simulink model "Simulink_asserv_Disc_21Mars_V2023b"  (R2023b)
settings: Solver=ode45  StartTime=0.0  StopTime=2500  FixedStep=0.01  RelTol=1e-3
model workspace (MAT data in the model file):
  AmbiantTemp = 23
  CondSig_mesureTemp_Gain = 3.3
  CondSig_mesureTemp_Vsub = 1.85
  DivTen_mesureTemp_R_pullup = 10000
  DivTen_mesureTemp_Vcc = 5
  Estimateur_alpha = 0.5
  Filtre_mesureTemp_deno = [0.0033 1]
  Gain_Comparateur_VoltageControle = 0.32
  RC_deno = [3.22e-08 3.04e-05 0.00955 1]
  Sig = Simulink.Signal
  Sig.DataType = 'auto'
  Sig.Dimensions = -1
  Sig.DimensionsMode = 'auto'
  Sig.Complexity = 'auto'
  Sig.SampleTime = -1
  Sig.SamplingMode = 'auto'
  SourceCourant_Gain_Vcontrole_vers_A = 3.1564
  ThermoRes_SHTEMP_A = 0.003354
  ThermoRes_SHTEMP_B = 0.00026
  ThermoRes_SHTEMP_C = 1.6e-06
  ThermoRes_SHTEMP_D = 6.3e-08
  ThermoRes_SH_A = -14.65719
  ThermoRes_SH_B = 4798.842
  ThermoRes_SH_C = -115334
  ThermoRes_SH_D = -3730535
  ThermoRes_SH_R_nom = 10000
  periodeEchant = 2
  periodeEchant_temp = 0.5
  setupDelay = 4
libraries: simulink x1
settings Model: SimulationMode=rapid-accelerator  Creator=alcot161  LastModifiedBy=alcot161
settings RTWCC: GPUComputeCapability=5.0

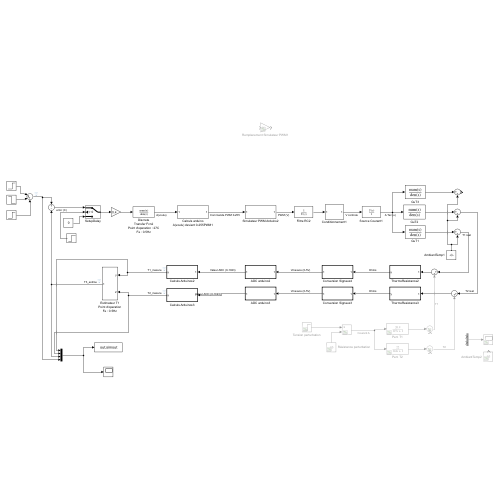
[thumbnail: Simulink's stored preview of the top-level diagram]
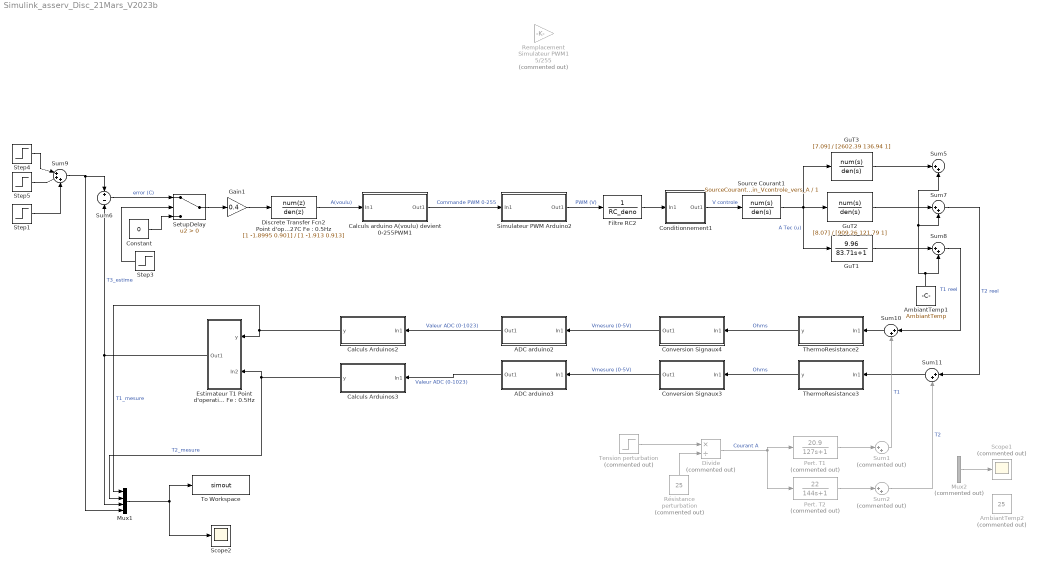
== system Simulink_asserv_Disc_21Mars_V2023b ==
  ADC arduino2 : Subsystem  TreatAsAtomicUnit=on
  ADC arduino3 : Subsystem  TreatAsAtomicUnit=on
  AmbiantTemp1 : Constant  Value=AmbiantTemp
  AmbiantTemp2 : Constant  Commented=on  Value=25
  Calculs Arduinos2 : Subsystem  TreatAsAtomicUnit=on
  Calculs Arduinos3 : Subsystem  TreatAsAtomicUnit=on
  Calculs arduino A(voulu) devient 0-255PWM1 : Subsystem
  Conditionnement1 : Subsystem
  Constant : Constant  Value=0  SampleTime=periodeEchant
  Conversion Signaux3 : Subsystem  TreatAsAtomicUnit=on
  Conversion Signaux4 : Subsystem  TreatAsAtomicUnit=on
  "Discrete Transfer Fcn2 Point d'operation : 27C Fe : 0.5Hz" : DiscreteTransferFcn  Numerator=[1 -1.8995 0.901]  Denominator=[1 -1.913 0.913]
  Divide : Product  Commented=on  Inputs=*/
  "Estimateur T1 Point d'operation Fe : 0.5Hz" : Subsystem
  Filtre RC2 : TransferFcn  Denominator=RC_deno
  Gain1 : Gain  Gain=0.4
  GuT1 : TransferFcn  Numerator=[9.96]  Denominator=[83.71 1]
  GuT2 : TransferFcn  Numerator=[8.07]  Denominator=[909.26 121.79 1]
  GuT3 : TransferFcn  Numerator=[7.09]  Denominator=[2602.39 136.94 1]
  Mux1 : Mux
  Mux2 : Mux  Commented=on  Inputs=2
  Pert. T1 : TransferFcn  Commented=on  Numerator=[20.9]  Denominator=[127 1]
  Pert. T2 : TransferFcn  Commented=on  Numerator=[22]  Denominator=[144 1]
  Remplacement Simulateur PWM1 : Gain  Commented=on  Gain=5/255
  Résistance perturbation : Constant  Commented=on  Value=25
  Scope1 : Scope  Commented=on
  Scope2 : Scope
  SetupDelay : Switch  Criteria=u2 > Threshold  SaturateOnIntegerOverflow=off  InputSameDT=off
  Simulateur PWM Arduino2 : Subsystem
  Source Courant1 : TransferFcn  Numerator=SourceCourant_Gain_Vcontrole_vers_A  Denominator=1
  Step1 : Step  Time=2130  After=3  SampleTime=0.05
  Step3 : Step  Time=setupDelay+1  SampleTime=periodeEchant
  Step4 : Step  Time=640  Before=AmbiantTemp  After=30  SampleTime=0.05
  Step5 : Step  Time=1290  After=-10  SampleTime=0.05
  Sum1 : Sum  Commented=on  Inputs=|++
  Sum{5,7..8,10..11} (5 alike) : Sum  Inputs=|++
  Sum2 : Sum  Commented=on  Inputs=|++
  Sum6 : Sum  Inputs=+|-  SampleTime=periodeEchant
  Sum9 : Sum  Inputs=|+++
  Tension perturbation : Step  Commented=on  Time=500  After=5  SampleTime=0.05
  ThermoResistance2 : Subsystem  TreatAsAtomicUnit=on
  ThermoResistance3 : Subsystem  TreatAsAtomicUnit=on
  To Workspace : ToWorkspace  VariableName=simout  SaveFormat=Timeseries  SampleTime=-1
  wires:
  ThermoResistance3/1(y) -> Conversion Signaux3/1(In1)  "Ohms"
  Step4/1 -> Sum9/1
  GuT2/1 -> Sum7/1
  Conversion Signaux3/1(Out1) -> ADC arduino3/1(In1)  "Vmesure (0-5V)"
  Sum9/1 -> Mux1/4, Sum6/1
  ADC arduino3/1(Out1) -> Calculs Arduinos3/1(In1)  "Valeur ADC (0-1023)"
  Simulateur PWM Arduino2/1(Out1) -> Filtre RC2/1  "PWM (V)"
  Step5/1 -> Sum9/2
  Conversion Signaux4/1(Out1) -> ADC arduino2/1(In1)  "Vmesure (0-5V)"
  AmbiantTemp1/1 -> Sum5/2, Sum7/2, Sum8/2
  Filtre RC2/1 -> Conditionnement1/1(In1)
  Calculs Arduinos2/1(y) -> Mux1/1, "Estimateur T1 Point d'operation Fe : 0.5Hz"/1(y)  "T1_mesure"
  ADC arduino2/1(Out1) -> Calculs Arduinos2/1(In1)  "Valeur ADC (0-1023)"
  Calculs arduino A(voulu) devient 0-255PWM1/1(Out1) -> Simulateur PWM Arduino2/1(In1)  "Commande PWM 0-255"
  Calculs Arduinos3/1(y) -> Mux1/2, "Estimateur T1 Point d'operation Fe : 0.5Hz"/2(In2)  "T2_mesure"
  Source Courant1/1 -> GuT3/1, GuT2/1, GuT1/1  "A Tec (u)"
  ThermoResistance2/1(y) -> Conversion Signaux4/1(In1)  "Ohms"
  Sum7/1 -> Sum11/1  "T2 reel"
  Conditionnement1/1(Out1) -> Source Courant1/1  "V controle"
  GuT1/1 -> Sum8/1
  GuT3/1 -> Sum5/1
  "Discrete Transfer Fcn2 Point d'operation : 27C Fe : 0.5Hz"/1 -> Calculs arduino A(voulu) devient 0-255PWM1/1(In1)  "A(voulu)"
  "Estimateur T1 Point d'operation Fe : 0.5Hz"/1(Out1) -> Mux1/3, Sum6/2  "T3_estime"
  Step3/1 -> SetupDelay/2
  Gain1/1 -> "Discrete Transfer Fcn2 Point d'operation : 27C Fe : 0.5Hz"/1
  Sum6/1 -> SetupDelay/1  "error (C)"
  SetupDelay/1 -> Gain1/1
  Constant/1 -> SetupDelay/3
  Sum8/1 -> Sum10/1  "T1 reel"
  Sum10/1 -> ThermoResistance2/1(In1)
  Sum11/1 -> ThermoResistance3/1(In1)
  Step1/1 -> Sum9/3
  Résistance perturbation/1 -> Divide/2
  Tension perturbation/1 -> Divide/1
  Divide/1 -> Pert. T2/1, Pert. T1/1  "Courant A"
  Sum1/1 -> Sum10/2  "T1"
  Sum2/1 -> Sum11/2  "T2"
  Pert. T1/1 -> Sum1/1
  Pert. T2/1 -> Sum2/1
  Mux2/1 -> Scope1/1
  Mux1/1 -> To Workspace/1, Scope2/1

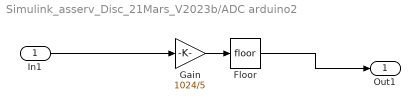
== system Simulink_asserv_Disc_21Mars_V2023b/ADC arduino2 ==
  In1 : Inport
  Floor : Rounding
  Gain : Gain  Gain=1024/5
  Out1 : Outport  SampleTime=periodeEchant_temp
  wires:
  In1/1 -> Gain/1
  Gain/1 -> Floor/1
  Floor/1 -> Out1/1

== system Simulink_asserv_Disc_21Mars_V2023b/ADC arduino3 ==
  In1 : Inport
  Floor : Rounding
  Gain : Gain  Gain=1024/5
  Out1 : Outport  SampleTime=periodeEchant_temp
  wires:
  In1/1 -> Gain/1
  Gain/1 -> Floor/1
  Floor/1 -> Out1/1

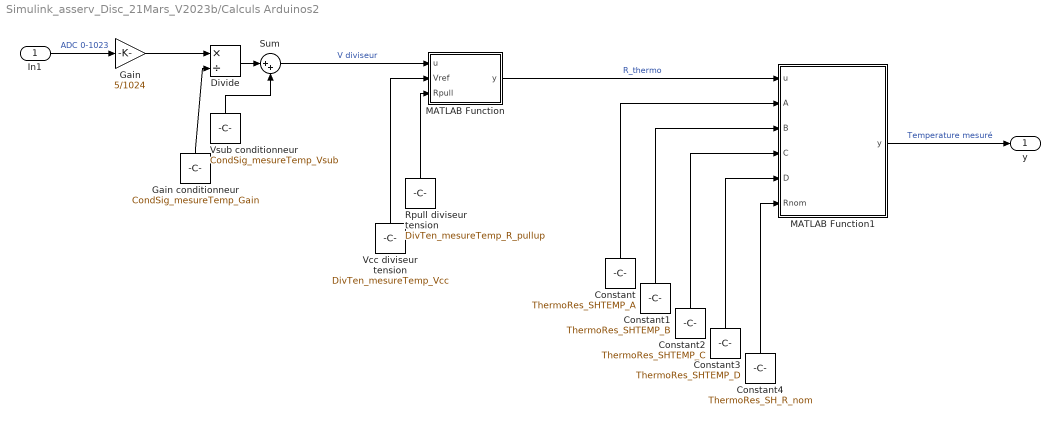
== system Simulink_asserv_Disc_21Mars_V2023b/Calculs Arduinos2 ==
  In1 : Inport
  Constant : Constant  Value=ThermoRes_SHTEMP_A
  Constant1 : Constant  Value=ThermoRes_SHTEMP_B
  Constant2 : Constant  Value=ThermoRes_SHTEMP_C
  Constant3 : Constant  Value=ThermoRes_SHTEMP_D
  Constant4 : Constant  Value=ThermoRes_SH_R_nom
  Divide : Product  Inputs=*/
  Gain : Gain  Gain=5/1024
  Gain conditionneur : Constant  Value=CondSig_mesureTemp_Gain
  MATLAB Function : MATLAB Function  TreatAsAtomicUnit=on
  MATLAB Function1 : MATLAB Function  TreatAsAtomicUnit=on
  Rpull diviseur tension : Constant  Value=DivTen_mesureTemp_R_pullup
  Sum : Sum  Inputs=|++
  Vcc diviseur tension : Constant  Value=DivTen_mesureTemp_Vcc
  Vsub conditionneur : Constant  Value=CondSig_mesureTemp_Vsub
  y : Outport
  wires:
  In1/1 -> Gain/1  "ADC 0-1023"
  Gain/1 -> Divide/1
  Gain conditionneur/1 -> Divide/2
  Divide/1 -> Sum/1
  Vsub conditionneur/1 -> Sum/2
  Sum/1 -> MATLAB Function/1(u)  "V diviseur"
  Rpull diviseur tension/1 -> MATLAB Function/3(Rpull)
  Vcc diviseur tension/1 -> MATLAB Function/2(Vref)
  MATLAB Function/1(y) -> MATLAB Function1/1(u)  "R_thermo"
  Constant/1 -> MATLAB Function1/2(A)
  Constant1/1 -> MATLAB Function1/3(B)
  Constant2/1 -> MATLAB Function1/4(C)
  Constant3/1 -> MATLAB Function1/5(D)
  Constant4/1 -> MATLAB Function1/6(Rnom)
  MATLAB Function1/1(y) -> y/1  "Temperature mesuré"

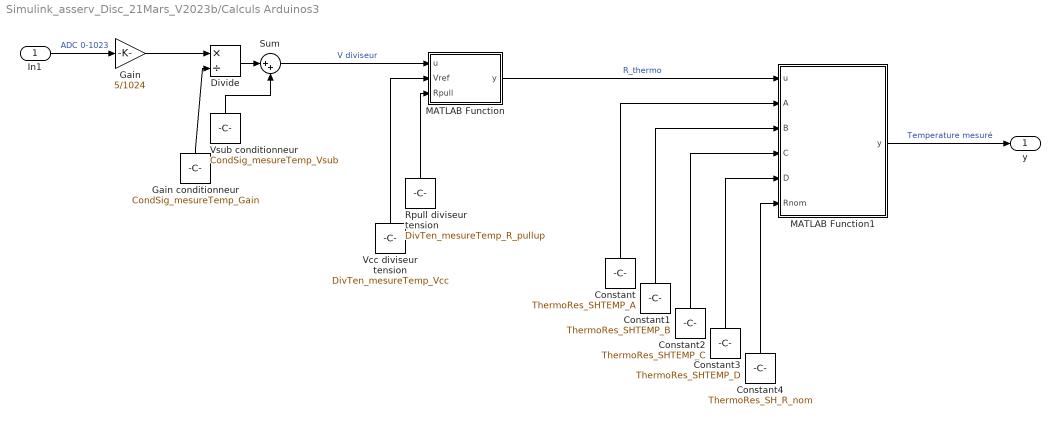
== system Simulink_asserv_Disc_21Mars_V2023b/Calculs Arduinos3 ==
  In1 : Inport
  Constant : Constant  Value=ThermoRes_SHTEMP_A
  Constant1 : Constant  Value=ThermoRes_SHTEMP_B
  Constant2 : Constant  Value=ThermoRes_SHTEMP_C
  Constant3 : Constant  Value=ThermoRes_SHTEMP_D
  Constant4 : Constant  Value=ThermoRes_SH_R_nom
  Divide : Product  Inputs=*/
  Gain : Gain  Gain=5/1024
  Gain conditionneur : Constant  Value=CondSig_mesureTemp_Gain
  MATLAB Function : MATLAB Function  TreatAsAtomicUnit=on
  MATLAB Function1 : MATLAB Function  TreatAsAtomicUnit=on
  Rpull diviseur tension : Constant  Value=DivTen_mesureTemp_R_pullup
  Sum : Sum  Inputs=|++
  Vcc diviseur tension : Constant  Value=DivTen_mesureTemp_Vcc
  Vsub conditionneur : Constant  Value=CondSig_mesureTemp_Vsub
  y : Outport
  wires:
  In1/1 -> Gain/1  "ADC 0-1023"
  Gain/1 -> Divide/1
  Gain conditionneur/1 -> Divide/2
  Divide/1 -> Sum/1
  Vsub conditionneur/1 -> Sum/2
  Sum/1 -> MATLAB Function/1(u)  "V diviseur"
  Rpull diviseur tension/1 -> MATLAB Function/3(Rpull)
  Vcc diviseur tension/1 -> MATLAB Function/2(Vref)
  MATLAB Function/1(y) -> MATLAB Function1/1(u)  "R_thermo"
  Constant/1 -> MATLAB Function1/2(A)
  Constant1/1 -> MATLAB Function1/3(B)
  Constant2/1 -> MATLAB Function1/4(C)
  Constant3/1 -> MATLAB Function1/5(D)
  Constant4/1 -> MATLAB Function1/6(Rnom)
  MATLAB Function1/1(y) -> y/1  "Temperature mesuré"

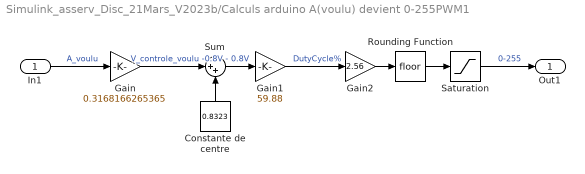
== system Simulink_asserv_Disc_21Mars_V2023b/Calculs arduino A(voulu) devient 0-255PWM1 ==
  In1 : Inport
  Constante de centre : Constant  Value=0.8323
  Gain : Gain  Gain=0.3168166265365
  Gain1 : Gain  Gain=59.88
  Gain2 : Gain  Gain=2.56  ParamMin=0  ParamMax=255.9  OutMin=[0]  OutMax=[255]
  Rounding Function : Rounding
  Saturation : Saturate  UpperLimit=255  LowerLimit=0  LinearizeAsGain=off
  Sum : Sum  Inputs=|++
  Out1 : Outport
  wires:
  In1/1 -> Gain/1  "A_voulu"
  Gain/1 -> Sum/1  "V_controle_voulu -0.8V - 0.8V"
  Sum/1 -> Gain1/1
  Constante de centre/1 -> Sum/2
  Gain1/1 -> Gain2/1  "DutyCycle%"
  Gain2/1 -> Rounding Function/1
  Rounding Function/1 -> Saturation/1
  Saturation/1 -> Out1/1  "0-255"

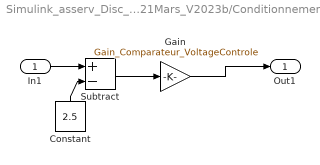
== system Simulink_asserv_Disc_21Mars_V2023b/Conditionnement1 ==
  In1 : Inport
  Constant : Constant  Value=2.5
  Gain : Gain  Gain=Gain_Comparateur_VoltageControle
  Subtract : Sum  Inputs=+-
  Out1 : Outport
  wires:
  In1/1 -> Subtract/1
  Constant/1 -> Subtract/2
  Subtract/1 -> Gain/1
  Gain/1 -> Out1/1

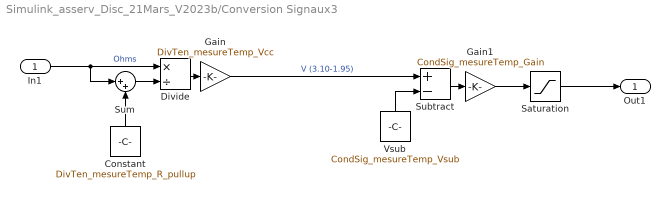
== system Simulink_asserv_Disc_21Mars_V2023b/Conversion Signaux3 ==
  In1 : Inport
  Constant : Constant  Value=DivTen_mesureTemp_R_pullup
  Divide : Product  Inputs=*/
  Gain : Gain  Gain=DivTen_mesureTemp_Vcc
  Gain1 : Gain  Gain=CondSig_mesureTemp_Gain
  Saturation : Saturate  UpperLimit=5  LowerLimit=0
  Subtract : Sum  Inputs=+-
  Sum : Sum  Inputs=|++
  Vsub : Constant  Value=CondSig_mesureTemp_Vsub
  Out1 : Outport
  wires:
  In1/1 -> Sum/1, Divide/1  "Ohms"
  Sum/1 -> Divide/2
  Constant/1 -> Sum/2
  Divide/1 -> Gain/1
  Vsub/1 -> Subtract/2
  Subtract/1 -> Gain1/1
  Gain1/1 -> Saturation/1
  Saturation/1 -> Out1/1
  Gain/1 -> Subtract/1  "V (3.10-1.95)"

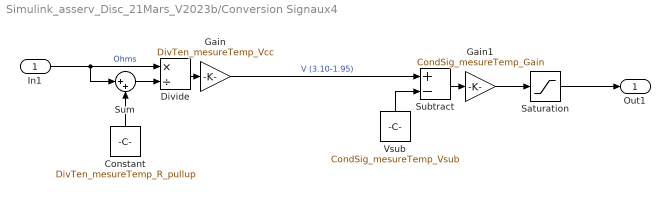
== system Simulink_asserv_Disc_21Mars_V2023b/Conversion Signaux4 ==
  In1 : Inport
  Constant : Constant  Value=DivTen_mesureTemp_R_pullup
  Divide : Product  Inputs=*/
  Gain : Gain  Gain=DivTen_mesureTemp_Vcc
  Gain1 : Gain  Gain=CondSig_mesureTemp_Gain
  Saturation : Saturate  UpperLimit=5  LowerLimit=0
  Subtract : Sum  Inputs=+-
  Sum : Sum  Inputs=|++
  Vsub : Constant  Value=CondSig_mesureTemp_Vsub
  Out1 : Outport
  wires:
  In1/1 -> Sum/1, Divide/1  "Ohms"
  Sum/1 -> Divide/2
  Constant/1 -> Sum/2
  Divide/1 -> Gain/1
  Vsub/1 -> Subtract/2
  Subtract/1 -> Gain1/1
  Gain1/1 -> Saturation/1
  Saturation/1 -> Out1/1
  Gain/1 -> Subtract/1  "V (3.10-1.95)"

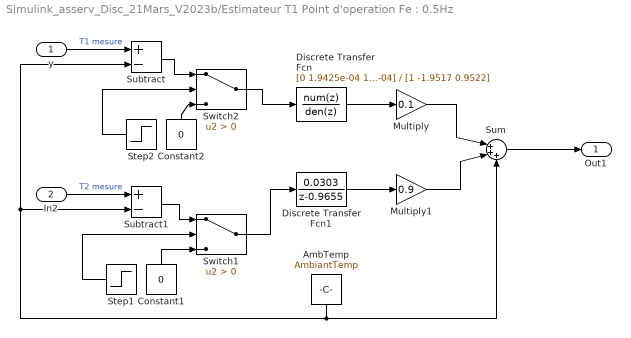
== system Simulink_asserv_Disc_21Mars_V2023b/Estimateur T1 Point d'operation Fe : 0.5Hz ==
  y : Inport
  In2 : Inport  Port=2
  AmbTemp : Constant  Value=AmbiantTemp  SampleTime=periodeEchant_temp
  Constant1 : Constant  Value=0  SampleTime=2
  Constant2 : Constant  Value=0  SampleTime=2
  Discrete Transfer Fcn : DiscreteTransferFcn  Numerator=[0 1.9425e-04 1.9111e-04]  Denominator=[1 -1.9517 0.9522]
  Discrete Transfer Fcn1 : DiscreteTransferFcn  Numerator=[0 0.0303]  Denominator=[1 -0.9655]
  Multiply : Gain  Gain=0.1
  Multiply1 : Gain  Gain=0.9
  Step1 : Step  Time=setupDelay  SampleTime=periodeEchant
  Step2 : Step  Time=setupDelay  SampleTime=periodeEchant
  Subtract : Sum  Inputs=+-
  Subtract1 : Sum  Inputs=+-
  Sum : Sum  Inputs=|+++
  Switch1 : Switch  Criteria=u2 > Threshold  SaturateOnIntegerOverflow=off  InputSameDT=off
  Switch2 : Switch  Criteria=u2 > Threshold  SaturateOnIntegerOverflow=off  InputSameDT=off
  Out1 : Outport  SampleTime=periodeEchant_temp
  wires:
  In2/1 -> Subtract1/1  "T2 mesure"
  Multiply/1 -> Sum/1
  Multiply1/1 -> Sum/2
  y/1 -> Subtract/1  "T1 mesure"
  Sum/1 -> Out1/1
  Discrete Transfer Fcn/1 -> Multiply/1
  Discrete Transfer Fcn1/1 -> Multiply1/1
  AmbTemp/1 -> Subtract/2, Subtract1/2, Sum/3
  Constant1/1 -> Switch1/3
  Constant2/1 -> Switch2/3
  Step2/1 -> Switch2/2
  Subtract/1 -> Switch2/1
  Switch2/1 -> Discrete Transfer Fcn/1
  Subtract1/1 -> Switch1/1
  Step1/1 -> Switch1/2
  Switch1/1 -> Discrete Transfer Fcn1/1

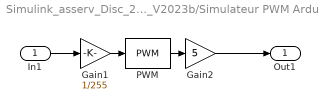
== system Simulink_asserv_Disc_21Mars_V2023b/Simulateur PWM Arduino2 ==
  In1 : Inport
  Gain1 : Gain  Gain=1/255
  Gain2 : Gain  Gain=5
  PWM : simulink/Discontinuities/PWM  DisableCoverage=on  Period=0.00204  InitialDelay=0  DisallowZeroDutyCycle=off  RunAtFixedTimeIntervals=off  SampleTime=0.1
  Out1 : Outport
  wires:
  Gain1/1 -> PWM/1
  PWM/1 -> Gain2/1
  In1/1 -> Gain1/1
  Gain2/1 -> Out1/1

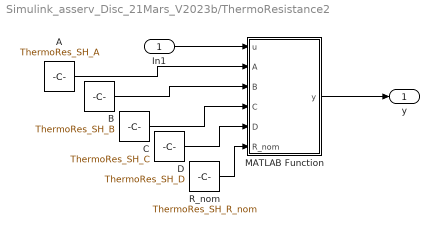
== system Simulink_asserv_Disc_21Mars_V2023b/ThermoResistance2 ==
  In1 : Inport
  A : Constant  Value=ThermoRes_SH_A
  B : Constant  Value=ThermoRes_SH_B
  C : Constant  Value=ThermoRes_SH_C
  D : Constant  Value=ThermoRes_SH_D
  MATLAB Function : MATLAB Function  TreatAsAtomicUnit=on
  R_nom : Constant  Value=ThermoRes_SH_R_nom
  y : Outport
  wires:
  In1/1 -> MATLAB Function/1(u)
  MATLAB Function/1(y) -> y/1
  A/1 -> MATLAB Function/2(A)
  B/1 -> MATLAB Function/3(B)
  C/1 -> MATLAB Function/4(C)
  D/1 -> MATLAB Function/5(D)
  R_nom/1 -> MATLAB Function/6(R_nom)

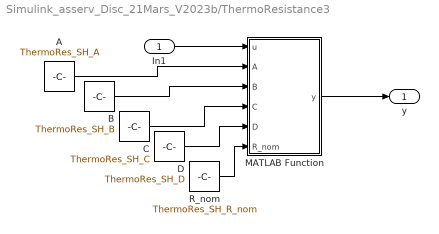
== system Simulink_asserv_Disc_21Mars_V2023b/ThermoResistance3 ==
  In1 : Inport
  A : Constant  Value=ThermoRes_SH_A
  B : Constant  Value=ThermoRes_SH_B
  C : Constant  Value=ThermoRes_SH_C
  D : Constant  Value=ThermoRes_SH_D
  MATLAB Function : MATLAB Function  TreatAsAtomicUnit=on
  R_nom : Constant  Value=ThermoRes_SH_R_nom
  y : Outport
  wires:
  In1/1 -> MATLAB Function/1(u)
  MATLAB Function/1(y) -> y/1
  A/1 -> MATLAB Function/2(A)
  B/1 -> MATLAB Function/3(B)
  C/1 -> MATLAB Function/4(C)
  D/1 -> MATLAB Function/5(D)
  R_nom/1 -> MATLAB Function/6(R_nom)

== matlab function Simulink_asserv_Disc_21Mars_V2023b/Calculs Arduinos2/MATLAB Function ==
  data: u input; y output; Vref input; Rpull input
function y = fcn(u, Vref, Rpull)

y = Rpull * (u/(Vref-u));

== matlab function Simulink_asserv_Disc_21Mars_V2023b/Calculs Arduinos2/MATLAB Function1 ==
  data: u input; y output; A input; B input; C input; D input; Rnom input
function y = fcn(u, A, B, C, D, Rnom)
    invT = A + B*log(u/Rnom) + C*(log(u/Rnom))^2 + D*(log(u/Rnom))^3;
    T = (1/invT) - 273.15;
y = T;

== matlab function Simulink_asserv_Disc_21Mars_V2023b/Calculs Arduinos3/MATLAB Function ==
  data: u input; y output; Vref input; Rpull input
function y = fcn(u, Vref, Rpull)

y = Rpull * (u/(Vref-u));

== matlab function Simulink_asserv_Disc_21Mars_V2023b/Calculs Arduinos3/MATLAB Function1 ==
  data: u input; y output; A input; B input; C input; D input; Rnom input
function y = fcn(u, A, B, C, D, Rnom)
    invT = A + B*log(u/Rnom) + C*(log(u/Rnom))^2 + D*(log(u/Rnom))^3;
    T = (1/invT) - 273.15;
y = T;

== matlab function Simulink_asserv_Disc_21Mars_V2023b/ThermoResistance2/MATLAB Function ==
  data: u input; y output; A input; B input; C input; D input; R_nom input
function y = fcn(u, A, B, C, D, R_nom)
   
y = R_nom * exp(A + (B/(u+273.15)) + (C/((u + 273.15)^2)) + (D/((u + 273.15)^3)));

== matlab function Simulink_asserv_Disc_21Mars_V2023b/ThermoResistance3/MATLAB Function ==
  data: u input; y output; A input; B input; C input; D input; R_nom input
function y = fcn(u, A, B, C, D, R_nom)
   
y = R_nom * exp(A + (B/(u+273.15)) + (C/((u + 273.15)^2)) + (D/((u + 273.15)^3)));
